simulink model "ThdRwLtStCshnFldCtrl"  (R2024b)
settings: Solver=FixedStepDiscrete  StartTime=0.0  StopTime=10.0  FixedStep=0.01  RelTol=1e-3
undefined symbols (not defined in the file or in its folder): KeSMSuMdMotFinshdTm_Val, KeSMSuMdRetryTm1_Val, KeSMSuModeReqDurgTm_Val
libraries: StCtrlLib x1
settings Model: Creator=sn2xws  LastModifiedBy=sn55gm
settings SolverCC: AlgebraicLoopSolver=TrustRegion
settings DataIOCC: SaveFormat=StructureWithTime  ReturnWorkspaceOutputs=off
settings OptimizationCC: DefaultParameterBehavior=Inlined  EnhancedBackFolding=on  PassReuseOutputArgsAs=Individual arguments  ZeroExternalMemoryAtStartup=off  ZeroInternalMemoryAtStartup=off  OptimizeBlockOrder=speed  DifferentSizesBufferReuse=on  OptimizationCustomize=off  EfficientTunableParamExpr=on
settings DebuggingCC: ParameterTunabilityLossMsg=error  UnconnectedInputMsg=warning  UnconnectedOutputMsg=warning  UnconnectedLineMsg=warning  ArithmeticOperatorsInVariantConditions=warning
settings ModelReferenceCC: EnableRefExpFcnMdlSchedulingChecks=on  ModelReferenceNumInstancesAllowed=Single
settings SFSimCC: MATLABDynamicMemAlloc=off  CustomCodeUndefinedFunction=UseInterfaceOnly
settings RTWCC: Description=AUTOSAR  SystemTargetFile=autosar.tlc  GenCodeOnly=on  TemplateMakefile=ert_default_tmf  GenerateReport=on  IncludeHyperlinkInReport=on  LaunchReport=on  DataTypeReplacement=CDataTypesFixedWidth  GenerateTraceInfo=on  GenerateTraceReport=on  GenerateTraceReportSl=on  GenerateTraceReportSf=on  GenerateTraceReportEml=on  GPUComputeCapability=3.5
settings CodeAppCC: ForceParamTrailComments=on  IgnoreCustomStorageClasses=off  OperatorAnnotations=on  SimulinkDataObjDesc=on  SFDataObjDesc=on  InsertBlockDesc=on
settings STFCustomTargetCC: TargetLangStandard=C99 (ISO)  MultiwordLength=256  ParMdlRefBuildCompliant=on  CompOptLevelCompliant=on  IncludeMdlTerminateFcn=off  CombineOutputUpdateFcns=on  SuppressErrorStatus=on  ERTCustomFileBanners=on  SupportNonFinite=off  SupportComplex=off  SupportContinuousTime=off  SupportNonInlinedSFcns=off  RemoveResetFunc=on  MATLABClassNameForMDSCustomization=Simulink.SoftwareTarget.ERTCustomization  AutosarCompliant=on  UseToolchainInfoCompliant=on  LookupTableObjectStructAxisOrder=2,1,3,4,...  LUTObjectStructOrderEvenSpacing=Size,Table,Breakpoints  SystemTargetFile=autosar.tlc
settings ERTTargetCC: TargetLangStandard=C99 (ISO)  ConcurrentExecutionCompliant=off  IncludeMdlTerminateFcn=off  SuppressErrorStatus=on  SupportNonFinite=off  SupportComplex=off  ModelStepFunctionPrototypeControlCompliant=off  CPPClassGenCompliant=off  AutosarCompliant=on  LookupTableObjectStructAxisOrder=2,1,3,4,...  LUTObjectStructOrderEvenSpacing=Size,Table,Breakpoints  ERTCustomFileTemplate=example_file_process.tlc  ERTFilePackagingFormat=Compact  BooleanTrueId=TRUE  BooleanFalseId=FALSE  DynamicArrayContainerType=coder::array

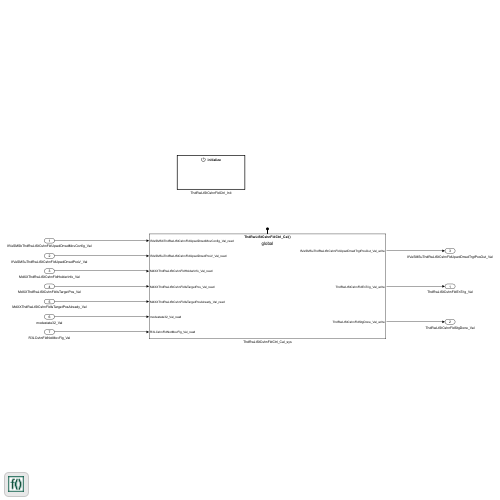
[thumbnail: Simulink's stored preview of the top-level diagram]
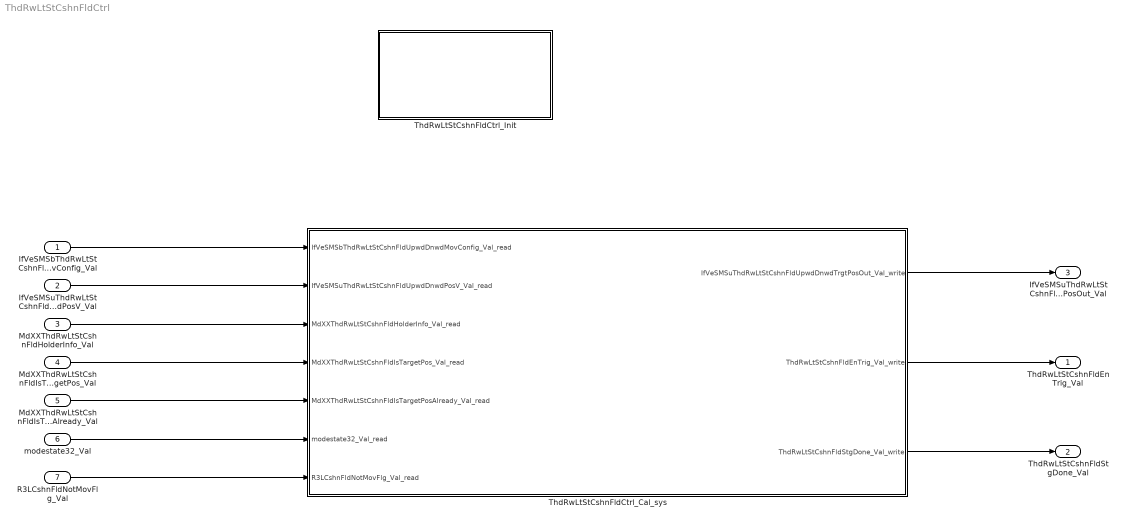
== system ThdRwLtStCshnFldCtrl ==
  IfVeSMSbThdRwLtStCshnFldUpwdDnwdMovConfig_Val : Inport  OutDataTypeStr=boolean  PortDimensions=1
  IfVeSMSuThdRwLtStCshnFldUpwdDnwdPosV_Val : Inport  Port=2  OutDataTypeStr=boolean  PortDimensions=1
  MdXXThdRwLtStCshnFldHolderInfo_Val : Inport  Port=3  OutDataTypeStr=uint32  PortDimensions=1
  MdXXThdRwLtStCshnFldIsTargetPos_Val : Inport  Port=4  OutDataTypeStr=uint32  PortDimensions=1
  MdXXThdRwLtStCshnFldIsTargetPosAlready_Val : Inport  Port=5  OutDataTypeStr=uint32  PortDimensions=1
  modestate32_Val : Inport  Port=6  OutDataTypeStr=uint32  PortDimensions=1
  R3LCshnFldNotMovFlg_Val : Inport  Port=7  OutDataTypeStr=boolean  PortDimensions=1
  ThdRwLtStCshnFldCtrl_Cal_sys : Subsystem
  ThdRwLtStCshnFldCtrl_Init : Subsystem
  ThdRwLtStCshnFldEnTrig_Val : Outport  OutDataTypeStr=boolean  PortDimensions=1  VectorParamsAs1DForOutWhenUnconnected=off
  ThdRwLtStCshnFldStgDone_Val : Outport  Port=2  OutDataTypeStr=boolean  PortDimensions=1  VectorParamsAs1DForOutWhenUnconnected=off
  IfVeSMSuThdRwLtStCshnFldUpwdDnwdTrgtPosOut_Val : Outport  Port=3  OutDataTypeStr=boolean  PortDimensions=1  VectorParamsAs1DForOutWhenUnconnected=off
  wires:
  IfVeSMSbThdRwLtStCshnFldUpwdDnwdMovConfig_Val/1 -> ThdRwLtStCshnFldCtrl_Cal_sys/1(IfVeSMSbThdRwLtStCshnFldUpwdDnwdMovConfig_Val_read)
  IfVeSMSuThdRwLtStCshnFldUpwdDnwdPosV_Val/1 -> ThdRwLtStCshnFldCtrl_Cal_sys/2(IfVeSMSuThdRwLtStCshnFldUpwdDnwdPosV_Val_read)
  MdXXThdRwLtStCshnFldHolderInfo_Val/1 -> ThdRwLtStCshnFldCtrl_Cal_sys/3(MdXXThdRwLtStCshnFldHolderInfo_Val_read)
  MdXXThdRwLtStCshnFldIsTargetPos_Val/1 -> ThdRwLtStCshnFldCtrl_Cal_sys/4(MdXXThdRwLtStCshnFldIsTargetPos_Val_read)
  MdXXThdRwLtStCshnFldIsTargetPosAlready_Val/1 -> ThdRwLtStCshnFldCtrl_Cal_sys/5(MdXXThdRwLtStCshnFldIsTargetPosAlready_Val_read)
  modestate32_Val/1 -> ThdRwLtStCshnFldCtrl_Cal_sys/6(modestate32_Val_read)
  R3LCshnFldNotMovFlg_Val/1 -> ThdRwLtStCshnFldCtrl_Cal_sys/7(R3LCshnFldNotMovFlg_Val_read)
  ThdRwLtStCshnFldCtrl_Cal_sys/1(IfVeSMSuThdRwLtStCshnFldUpwdDnwdTrgtPosOut_Val_write) -> IfVeSMSuThdRwLtStCshnFldUpwdDnwdTrgtPosOut_Val/1
  ThdRwLtStCshnFldCtrl_Cal_sys/2(ThdRwLtStCshnFldEnTrig_Val_write) -> ThdRwLtStCshnFldEnTrig_Val/1
  ThdRwLtStCshnFldCtrl_Cal_sys/3(ThdRwLtStCshnFldStgDone_Val_write) -> ThdRwLtStCshnFldStgDone_Val/1

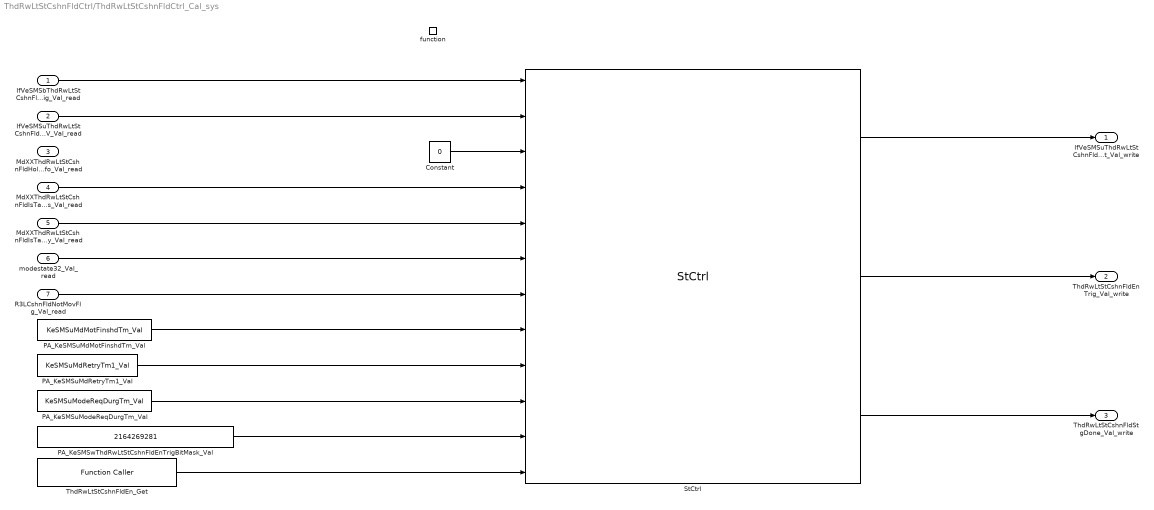
== system ThdRwLtStCshnFldCtrl/ThdRwLtStCshnFldCtrl_Cal_sys ==
  IfVeSMSbThdRwLtStCshnFldUpwdDnwdMovConfig_Val_read : Inport
  IfVeSMSuThdRwLtStCshnFldUpwdDnwdPosV_Val_read : Inport  Port=2
  MdXXThdRwLtStCshnFldHolderInfo_Val_read : Inport  Port=3
  MdXXThdRwLtStCshnFldIsTargetPos_Val_read : Inport  Port=4
  MdXXThdRwLtStCshnFldIsTargetPosAlready_Val_read : Inport  Port=5
  modestate32_Val_read : Inport  Port=6
  R3LCshnFldNotMovFlg_Val_read : Inport  Port=7
  function : TriggerPort  TriggerType=function-call  IsSimulinkFunction=on  FunctionName=ThdRwLtStCshnFldCtrl_Cal  VariantControl=(inherit)
  Constant : Constant  Value=0  OutDataTypeStr=uint32
  PA_KeSMSuMdMotFinshdTm_Val : Constant  Value=KeSMSuMdMotFinshdTm_Val
  PA_KeSMSuMdRetryTm1_Val : Constant  Value=KeSMSuMdRetryTm1_Val
  PA_KeSMSuModeReqDurgTm_Val : Constant  Value=KeSMSuModeReqDurgTm_Val
  PA_KeSMSwThdRwLtStCshnFldEnTrigBitMask_Val : Constant  Value=2164269281  OutDataTypeStr=uint32
  StCtrl : StCtrlLib/StCtrl  SystemSampleTime=-1  VariantActivationTime=update diagram  AllowFlexibleInterface=on  Latency=0  AutoFrameSizeCalculation=off
  ThdRwLtStCshnFldEn_Get : FunctionCaller  FunctionPrototype=data = ThdRwLtStCshnFldEn_Get()  InputArgumentSpecifications=<Enter example>  OutputArgumentSpecifications=uint32(1)
  IfVeSMSuThdRwLtStCshnFldUpwdDnwdTrgtPosOut_Val_write : Outport  VectorParamsAs1DForOutWhenUnconnected=off
      settings: EnsureOutportIsVirtual=on
  ThdRwLtStCshnFldEnTrig_Val_write : Outport  Port=2  VectorParamsAs1DForOutWhenUnconnected=off
      settings: EnsureOutportIsVirtual=on
  ThdRwLtStCshnFldStgDone_Val_write : Outport  Port=3  VectorParamsAs1DForOutWhenUnconnected=off
      settings: EnsureOutportIsVirtual=on
  wires:
  StCtrl/1 -> IfVeSMSuThdRwLtStCshnFldUpwdDnwdTrgtPosOut_Val_write/1
  StCtrl/2 -> ThdRwLtStCshnFldEnTrig_Val_write/1
  StCtrl/3 -> ThdRwLtStCshnFldStgDone_Val_write/1
  IfVeSMSuThdRwLtStCshnFldUpwdDnwdPosV_Val_read/1 -> StCtrl/2
  IfVeSMSbThdRwLtStCshnFldUpwdDnwdMovConfig_Val_read/1 -> StCtrl/1
  MdXXThdRwLtStCshnFldIsTargetPos_Val_read/1 -> StCtrl/4
  MdXXThdRwLtStCshnFldIsTargetPosAlready_Val_read/1 -> StCtrl/5
  modestate32_Val_read/1 -> StCtrl/6
  R3LCshnFldNotMovFlg_Val_read/1 -> StCtrl/7
  PA_KeSMSwThdRwLtStCshnFldEnTrigBitMask_Val/1 -> StCtrl/11
  ThdRwLtStCshnFldEn_Get/1 -> StCtrl/12
  PA_KeSMSuModeReqDurgTm_Val/1 -> StCtrl/10
  PA_KeSMSuMdMotFinshdTm_Val/1 -> StCtrl/8
  PA_KeSMSuMdRetryTm1_Val/1 -> StCtrl/9
  Constant/1 -> StCtrl/3

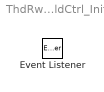
== system ThdRwLtStCshnFldCtrl/ThdRwLtStCshnFldCtrl_Init ==
  Event Listener : EventListener  EventName=reset
